simulink model "Deliverable1_SimulinkModel_Group33"  (R2023b)
settings: Solver=FixedStepAuto  StartTime=0.0  StopTime=10.0  RelTol=1e-3  EnableMultiTasking=on
undefined symbols (not defined in the file): D0, D1, D10, D11, D12, D13, D2, D3, D4, D5, D6, D7, D8, D9, PTA0, PTA1, PTA2, PTB23, PTB9, PTC16, PTC17, PTC2, PTC3, PTC4, PTD0, PTD1, PTD2, PTD3
libraries: frdmk64flib x14
settings Model: ExtModeTrigDuration=5  Creator=cakes  LastModifiedBy=cakes
settings OptimizationCC: EnhancedBackFolding=on  PassReuseOutputArgsAs=Individual arguments  ZeroExternalMemoryAtStartup=off  ZeroInternalMemoryAtStartup=off  MaxStackSize=64  OptimizeBlockOrder=speed  DifferentSizesBufferReuse=on  OptimizationCustomize=off  EfficientTunableParamExpr=on
settings DebuggingCC: ParameterTunabilityLossMsg=error
settings HardwareCC: ProdBitPerPointer=32  ProdBitPerSizeT=32  ProdBitPerPtrDiffT=32  ProdLargestAtomicInteger=Long  ProdLargestAtomicFloat=Double  ProdWordSize=32  ProdHWDeviceType=ARM Compatible->ARM Cortex
settings SFSimCC: MATLABDynamicMemAlloc=off
settings RTWCC: Description=Embedded Coder  SystemTargetFile=ert.tlc  HardwareBoard=NXP FRDM-K64F  TLCOptions="-aInlineSetEventsForThisBaseRateFcn=TLC_FALSE -aSuppressMultiTaskScheduler=TLC_FALSE  -aRateBasedStepFcn=0"  TemplateMakefile=ert_default_tmf  Toolchain=GNU Tools for ARM Embedded Processors
settings CodeAppCC: ForceParamTrailComments=on  IgnoreCustomStorageClasses=off  OperatorAnnotations=on  SimulinkDataObjDesc=on  SFDataObjDesc=on  InsertBlockDesc=on
settings ERTTargetCC: ExtModeTransport=4  ExtModeMexFile=sendToCommService

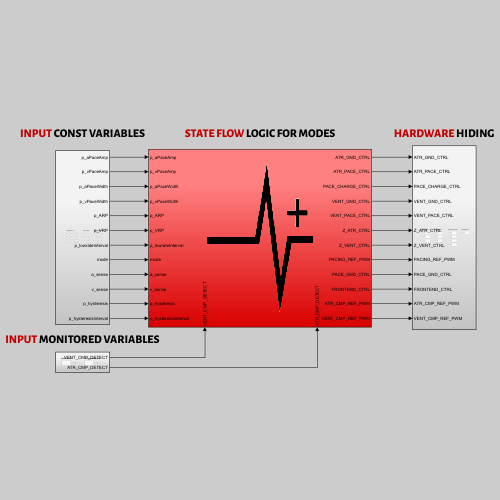
[thumbnail: Simulink's stored preview of the top-level diagram]
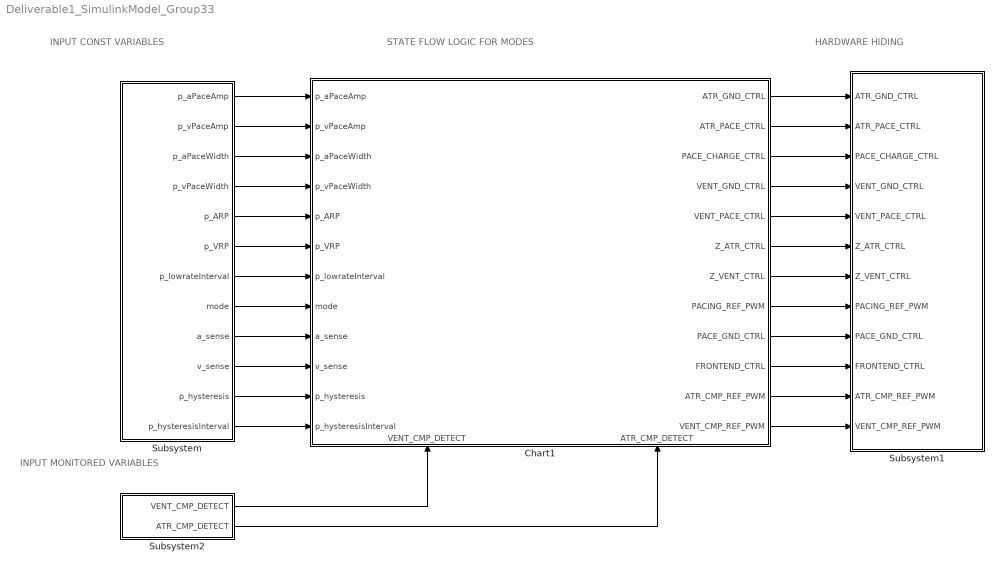
== system Deliverable1_SimulinkModel_Group33 ==
  note: STATE FLOW LOGIC FOR MODES
  note: INPUT CONST VARIABLES
  note: HARDWARE HIDING
  note: INPUT MONITORED VARIABLES
  Chart1 : Stateflow chart  TreatAsAtomicUnit=on
      settings: PortSchema="{\"entries\":[{\"content\":{\"sides\":[{\"content\":{\"connectorIds\":[\"In3\",\"In4\",\"In5\",\"In6\",\"In7\",\"In8\",\"In9\",\"In12\",\"In10\",\"In11\",\"In14\",\"In13\"]},\"type\":\"ConnectorPlacement.EquallySpacedRectSide\",\"uuid\":\"0645b224-ea0f-4252-ab3f-59541b69d578\"},{\"content\":{\"connectorIds\":[\"Out1\",\"Out2\",\"Out3\",\"Out4\",\"Out5\",\"Out6\",\"Out7\",\"Out8\",\"Out9\",\"Out10\",\"Out12\",\"Out11\"],\"side\":\"RIGHT\"},\"type\":\"ConnectorPlacement.EquallySpacedRectSide\",\"uuid\":\"774839c9-1eb4-4ab6-be6e-099c2bb8a485\"},{\"content\":{\"side\":\"TOP\"},\"type\":\"ConnectorPlacement.EquallySpacedRectSide\",\"uuid\":\"6cb60565-1780-4b9d-884d-75d2ba8c5024\"},{\"content\":{\"connectorIds\":[\"In1\",\"In2\"],\"side\":\"BOTTOM\"},\"type\":\"ConnectorPlacement.EquallySpacedRectSide\",\"uuid\":\"cb44bc08-16a9-4dba-a42a-7ec56f3e5fd4\"}]},\"type\":\"ConnectorPlacement.EquallySpacedConnector\",\"uuid\":\"755e29d5-bc4e-404e-b866-950d5e4fdc89\"}],\"packageUris\":[\"http://schema.mathworks.com/mf0/Connector/R2020b\"],\"version\":\"1.0\"}"
  Subsystem : Subsystem
  Subsystem1 : Subsystem
  Subsystem2 : Subsystem
  wires:
  Subsystem/1(p_aPaceAmp) -> Chart1/3(p_aPaceAmp)
  Subsystem/2(p_vPaceAmp) -> Chart1/4(p_vPaceAmp)
  Subsystem/3(p_aPaceWidth) -> Chart1/5(p_aPaceWidth)
  Subsystem/4(p_vPaceWidth) -> Chart1/6(p_vPaceWidth)
  Subsystem/5(p_ARP) -> Chart1/7(p_ARP)
  Subsystem/6(p_VRP) -> Chart1/8(p_VRP)
  Subsystem/7(p_lowrateInterval) -> Chart1/9(p_lowrateInterval)
  Subsystem/8(mode) -> Chart1/12(mode)
  Chart1/1(ATR_GND_CTRL) -> Subsystem1/1(ATR_GND_CTRL)
  Chart1/2(ATR_PACE_CTRL) -> Subsystem1/2(ATR_PACE_CTRL)
  Chart1/3(PACE_CHARGE_CTRL) -> Subsystem1/3(PACE_CHARGE_CTRL)
  Chart1/4(VENT_GND_CTRL) -> Subsystem1/4(VENT_GND_CTRL)
  Chart1/5(VENT_PACE_CTRL) -> Subsystem1/5(VENT_PACE_CTRL)
  Chart1/6(Z_ATR_CTRL) -> Subsystem1/6(Z_ATR_CTRL)
  Subsystem2/1(VENT_CMP_DETECT) -> Chart1/1(VENT_CMP_DETECT)
  Chart1/9(PACE_GND_CTRL) -> Subsystem1/9(PACE_GND_CTRL)
  Subsystem/9(a_sense) -> Chart1/10(a_sense)
  Subsystem/10(v_sense) -> Chart1/11(v_sense)
  Chart1/10(FRONTEND_CTRL) -> Subsystem1/10(FRONTEND_CTRL)
  Chart1/11(VENT_CMP_REF_PWM) -> Subsystem1/12(VENT_CMP_REF_PWM)
  Chart1/7(Z_VENT_CTRL) -> Subsystem1/7(Z_VENT_CTRL)
  Chart1/8(PACING_REF_PWM) -> Subsystem1/8(PACING_REF_PWM)
  Chart1/12(ATR_CMP_REF_PWM) -> Subsystem1/11(ATR_CMP_REF_PWM)
  Subsystem2/2(ATR_CMP_DETECT) -> Chart1/2(ATR_CMP_DETECT)
  Subsystem/11(p_hysteresis) -> Chart1/14(p_hysteresis)
  Subsystem/12(p_hysteresisInterval) -> Chart1/13(p_hysteresisInterval)

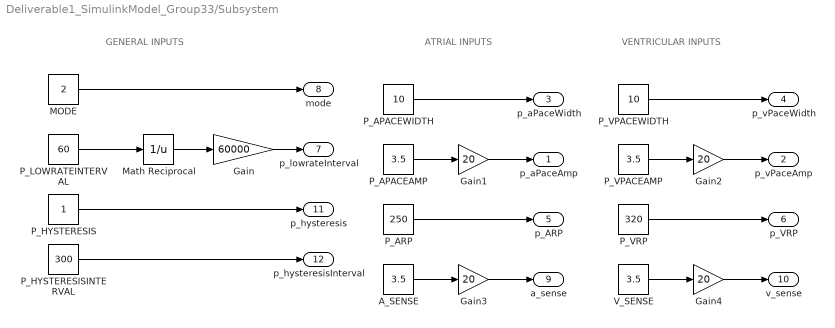
== system Deliverable1_SimulinkModel_Group33/Subsystem ==
  note: GENERAL INPUTS
  note: ATRIAL INPUTS
  note: VENTRICULAR INPUTS
  A_SENSE : Constant  Value=3.5
  Gain : Gain  Gain=60000
  Gain{1..4} (4 alike) : Gain  Gain=20
  MODE : Constant  Value=2
  Math Reciprocal : Math  Operator=reciprocal  SignedPower=on
  P_APACEAMP : Constant  Value=3.5
  P_APACEWIDTH : Constant  Value=10
  P_ARP : Constant  Value=250
  P_HYSTERESIS : Constant
  P_HYSTERESISINTERVAL : Constant  Value=300
  P_LOWRATEINTERVAL : Constant  Value=60
  P_VPACEAMP : Constant  Value=3.5
  P_VPACEWIDTH : Constant  Value=10
  P_VRP : Constant  Value=320
  V_SENSE : Constant  Value=3.5
  p_aPaceAmp : Outport
  p_vPaceAmp : Outport  Port=2
  p_aPaceWidth : Outport  Port=3
  p_vPaceWidth : Outport  Port=4
  p_ARP : Outport  Port=5
  p_VRP : Outport  Port=6
  p_lowrateInterval : Outport  Port=7
  mode : Outport  Port=8
  a_sense : Outport  Port=9
  v_sense : Outport  Port=10
  p_hysteresis : Outport  Port=11
  p_hysteresisInterval : Outport  Port=12
  wires:
  P_APACEWIDTH/1 -> p_aPaceWidth/1
  P_VPACEWIDTH/1 -> p_vPaceWidth/1
  MODE/1 -> mode/1
  P_ARP/1 -> p_ARP/1
  P_VRP/1 -> p_VRP/1
  P_HYSTERESIS/1 -> p_hysteresis/1
  P_HYSTERESISINTERVAL/1 -> p_hysteresisInterval/1
  P_LOWRATEINTERVAL/1 -> Math Reciprocal/1
  Math Reciprocal/1 -> Gain/1
  Gain/1 -> p_lowrateInterval/1
  P_APACEAMP/1 -> Gain1/1
  Gain1/1 -> p_aPaceAmp/1
  P_VPACEAMP/1 -> Gain2/1
  Gain2/1 -> p_vPaceAmp/1
  A_SENSE/1 -> Gain3/1
  V_SENSE/1 -> Gain4/1
  Gain4/1 -> v_sense/1
  Gain3/1 -> a_sense/1

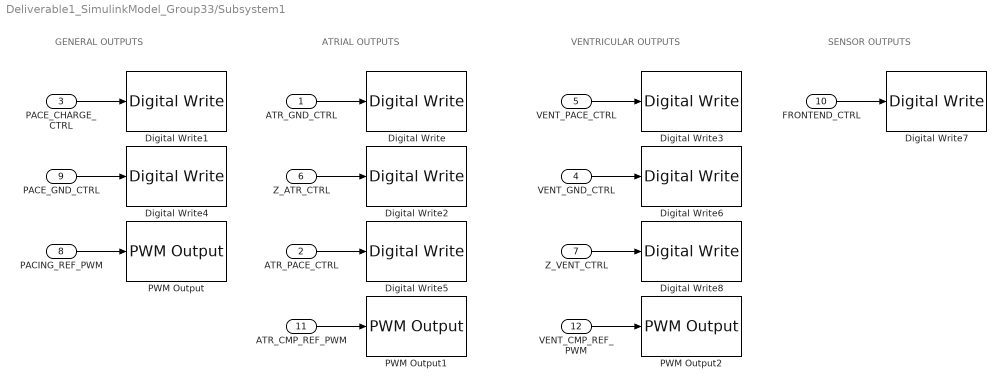
== system Deliverable1_SimulinkModel_Group33/Subsystem1 ==
  note: ATRIAL OUTPUTS
  note: GENERAL OUTPUTS
  note: VENTRICULAR OUTPUTS
  note: SENSOR OUTPUTS
  ATR_GND_CTRL : Inport
  ATR_PACE_CTRL : Inport  Port=2
  PACE_CHARGE_CTRL : Inport  Port=3
  VENT_GND_CTRL : Inport  Port=4
  VENT_PACE_CTRL : Inport  Port=5
  Z_ATR_CTRL : Inport  Port=6
  Z_VENT_CTRL : Inport  Port=7
  PACING_REF_PWM : Inport  Port=8
  PACE_GND_CTRL : Inport  Port=9
  FRONTEND_CTRL : Inport  Port=10
  ATR_CMP_REF_PWM : Inport  Port=11
  VENT_CMP_REF_PWM : Inport  Port=12
  Digital Write : frdmk64flib/Digital Write  Whichpin=PTD2 (D11)
  Digital Write1 : frdmk64flib/Digital Write  Whichpin=PTB9 (D2)
  Digital Write2 : frdmk64flib/Digital Write  Whichpin=PTB23 (D4)
  Digital Write3 : frdmk64flib/Digital Write  Whichpin=PTC4 (D9)
  Digital Write4 : frdmk64flib/Digital Write  Whichpin=PTD0 (D10)
  Digital Write5 : frdmk64flib/Digital Write  Whichpin=PTA0 (D8)
  Digital Write6 : frdmk64flib/Digital Write  Whichpin=PTD3 (D12)
  Digital Write7 : frdmk64flib/Digital Write  Whichpin=PTD1 (D13)
  Digital Write8 : frdmk64flib/Digital Write  Whichpin=PTC3 (D7)
  PWM Output : frdmk64flib/PWM Output  Whichpin=PTA2 (D5)  InitialFrequency=2000  InitialDutyCycle=0
  PWM Output1 : frdmk64flib/PWM Output  Whichpin=PTC2 (D6)  InitialFrequency=2000  InitialDutyCycle=0
  PWM Output2 : frdmk64flib/PWM Output  Whichpin=PTA1 (D3)  InitialFrequency=2000  InitialDutyCycle=0
  wires:
  PACING_REF_PWM/1 -> PWM Output/1
  Z_ATR_CTRL/1 -> Digital Write2/1
  PACE_CHARGE_CTRL/1 -> Digital Write1/1
  ATR_PACE_CTRL/1 -> Digital Write5/1
  ATR_GND_CTRL/1 -> Digital Write/1
  VENT_PACE_CTRL/1 -> Digital Write3/1
  VENT_GND_CTRL/1 -> Digital Write6/1
  FRONTEND_CTRL/1 -> Digital Write7/1
  Z_VENT_CTRL/1 -> Digital Write8/1
  PACE_GND_CTRL/1 -> Digital Write4/1
  ATR_CMP_REF_PWM/1 -> PWM Output1/1
  VENT_CMP_REF_PWM/1 -> PWM Output2/1

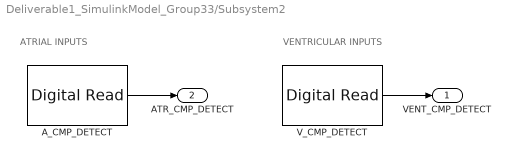
== system Deliverable1_SimulinkModel_Group33/Subsystem2 ==
  note: ATRIAL INPUTS
  note: VENTRICULAR INPUTS
  A_CMP_DETECT : frdmk64flib/Digital Read  Whichpin=PTC16 (D0)  SampleTime=0.001
  V_CMP_DETECT : frdmk64flib/Digital Read  Whichpin=PTC17 (D1)  SampleTime=0.001
  VENT_CMP_DETECT : Outport
  ATR_CMP_DETECT : Outport  Port=2
  wires:
  V_CMP_DETECT/1 -> VENT_CMP_DETECT/1
  A_CMP_DETECT/1 -> ATR_CMP_DETECT/1

== stateflow chart Deliverable1_SimulinkModel_Group33/Chart1 ==
  state INIT
    entry:
    %inital state, reset variables when mode change
    PACE_CHARGE_CTRL = 0;
    ATR_PACE_CTRL = 0;
    ATR_GND_CTRL = 0;
    VENT_PACE_CTRL=0;
    VENT_GND_CTRL=0;
    Z_ATR_CTRL = 0;
    Z_VENT_CTRL=0;
    PACE_GND_CTRL=0;
    PACING_REF_PWM=0;
    PACE_CHARGE_CTRL=0;
    FRONTEND_CTRL =0;
    VENT_CMP_REF_PWM = v_sense;
    ATR_CMP_REF_PWM = a_sense;
    note: MODE
        | NUMBER
        |
        | AOO
        | 0
        |
        | VOO
        | 1
        |
        | AAI
        | 2
        |
        | VVI
        | 3
  state AOO
    state AOO_Charging
      %charging capacitor
      entry:
      PACING_REF_PWM=p_aPaceAmp;
      PACE_GND_CTRL=1;
      Z_ATR_CTRL = 0;
      ATR_PACE_CTRL = 0;
      PACE_CHARGE_CTRL = 1;
      ATR_GND_CTRL = 1;
    state AOO_Pacing
      %discharging
      entry:
      Z_ATR_CTRL = 1;
      PACE_CHARGE_CTRL = 0;
      ATR_GND_CTRL = 0;
      ATR_PACE_CTRL = 1;
    (default) -> AOO_Charging
    AOO_Charging -> AOO_Pacing : after(p_lowrateInterval,msec)
    AOO_Pacing -> AOO_Charging : after(p_aPaceWidth,msec)
  state VOO
    state VOO_Charging
      %charging capacitor
      entry:
      PACING_REF_PWM=p_vPaceAmp;
      PACE_GND_CTRL=1;
      Z_VENT_CTRL = 0;
      VENT_PACE_CTRL = 0;
      PACE_CHARGE_CTRL = 1;
      VENT_GND_CTRL = 1;
    state VOO_Pacing
      %discharging capacitor
      entry:
      Z_VENT_CTRL = 1;
      PACE_CHARGE_CTRL = 0;
      VENT_GND_CTRL = 0;
      VENT_PACE_CTRL = 1;
    (default) -> VOO_Charging
    VOO_Charging -> VOO_Pacing : after(p_lowrateInterval,msec)
    VOO_Pacing -> VOO_Charging : after(p_vPaceWidth,msec)
  state AAI
    state pARP
      %atrial refractory period from paced beat
      entry:
      FRONTEND_CTRL = 1;
      PACING_REF_PWM = p_aPaceAmp;
      PACE_GND_CTRL=1;
      ATR_PACE_CTRL = 0;
      PACE_CHARGE_CTRL = 1;
      ATR_GND_CTRL = 1;
    state pReady
      %refratory period
      %finishes
    state Discharging
      %discharging
      entry:
      PACE_CHARGE_CTRL = 0;
      ATR_GND_CTRL = 0;
      ATR_PACE_CTRL = 1;
    state sARP
      %atrial refractory
      %period from
      %sensed beat
    state sReady
      %same as p-ready,
      %with period increased
      %if hysteresis is enabled
    AAI.Discharging -> pARP : after(p_aPaceWidth, msec)
    (default) -> pARP
    pARP -> AAI.pReady : after(p_ARP, msec)
    AAI.pReady -> AAI.Discharging [order 1] : after(p_lowrateInterval - p_ARP - p_aPaceWidth, msec)
    AAI.pReady -> sARP [order 2] : [ATR_CMP_DETECT]
    AAI.sReady -> AAI.Discharging [order 1] : after(p_lowrateInterval-p_ARP-p_aPaceWidth+(p_hysteresis*p_hysteresisInterval), msec)
    sARP -> AAI.sReady : after(p_ARP, msec)
    AAI.sReady -> sARP [order 2] : [ATR_CMP_DETECT]
  state VVI
    state pVRP
      %ventricular refractory period from paced beat
      entry:
      FRONTEND_CTRL = 1;
      PACING_REF_PWM = p_vPaceAmp;
      PACE_GND_CTRL=1;
      VENT_PACE_CTRL = 0;
      PACE_CHARGE_CTRL = 1;
      VENT_GND_CTRL = 1;
    state pReady
      %refratory period
      %finishes
    state Discharging
      %discharging
      entry:
      PACE_CHARGE_CTRL = 0;
      VENT_GND_CTRL = 0;
      VENT_PACE_CTRL = 1;
    state sVRP
      %atrial refractory
      %period from
      %sensed beat
    state sReady
      %same as p-ready,
      %with period increased
      %if hysteresis is enabled
    VVI.Discharging -> pVRP : after(p_vPaceWidth, msec)
    (default) -> pVRP
    pVRP -> VVI.pReady : after(p_VRP, msec)
    VVI.pReady -> VVI.Discharging [order 1] : after(p_lowrateInterval - p_VRP - p_vPaceWidth, msec)
    VVI.pReady -> sVRP [order 2] : [VENT_CMP_DETECT]
    VVI.sReady -> VVI.Discharging [order 1] : after(p_lowrateInterval-p_VRP-p_vPaceWidth+(p_hysteresis*p_hysteresisInterval), msec)
    sVRP -> VVI.sReady : after(p_VRP, msec)
    VVI.sReady -> sVRP [order 2] : [VENT_CMP_DETECT]
  INIT -> AOO [order 1] : [mode == 0]
  AOO -> INIT : [mode ~=0]
  VOO -> INIT : [mode~=1]
  INIT -> VOO [order 2] : [mode==1]
  (default) -> INIT
  AAI -> INIT : [mode ~=2]
  INIT -> AAI [order 3] : [mode == 2]
  INIT -> VVI [order 4] : [mode==3]
  VVI -> INIT : [mode~=3]
  data: VENT_CMP_DETECT input; ATR_CMP_DETECT input; ATR_GND_CTRL output; ATR_PACE_CTRL output; PACE_CHARGE_CTRL output; VENT_GND_CTRL output; VENT_PACE_CTRL output; Z_ATR_CTRL output; p_aPaceAmp input; p_vPaceAmp input; p_aPaceWidth input; p_vPaceWidth input; p_ARP input; p_VRP input; p_lowrateInterval input; a_sense input; v_sense input; mode input; Z_VENT_CTRL output; PACING_REF_PWM output; PACE_GND_CTRL output; FRONTEND_CTRL output; VENT_CMP_REF_PWM output; ATR_CMP_REF_PWM output; p_hysteresisInterval input; p_hysteresis input
